simulink model "example_PV_Generator_with_Inverter"  (R2018b)
settings: Solver=ode45  StartTime=0*24*3600  StopTime=24*3600  MaxStep=60  RelTol=1e-4  EnableMultiTasking=on
undefined symbols (not defined in the file): path_carnot
libraries: carnot x4
settings Model: Creator=drhf  LastModifiedBy=drhf
settings DataIOCC: LimitDataPoints=on  SaveFormat=Array  SignalLoggingSaveFormat=ModelDataLogs
settings OptimizationCC: ExpressionDepthLimit=2147483647  LifeSpan=inf
settings DebuggingCC: UnderspecifiedInitializationDetection=Classic  MergeDetectMultiDrivingBlocksExec=none  SolverPrmCheckMsg=warning  FcnCallInpInsideContextMsg=warning  StateNameClashWarn=warning  SFUnexpectedBacktrackingDiag=warning  SFNoUnconditionalDefaultTransitionDiag=warning  SFExecutionAtInitializationDiag=none
settings HardwareCC: ProdBitPerPointer=32  ProdBitPerSizeT=32  ProdBitPerPtrDiffT=32  ProdLargestAtomicFloat=None  ProdIntDivRoundTo=Undefined  ProdEndianess=Unspecified  ProdWordSize=32  ProdHWDeviceType=32-bit Generic
settings ModelReferenceCC: PropagateSignalLabelsOutOfModel=off
settings SFSimCC: SimUseLocalCustomCode=off
settings RTWCC: RTWUseLocalCustomCode=off
settings CodeAppCC: StateflowObjectComments=on
settings GRTTargetCC: TargetLangStandard=C89/C90 (ANSI)  GeneratePreprocessorConditionals=Disable all  CombineOutputUpdateFcns=off  GRTInterface=on
settings ConfigComp: CovMetricSettings=dw  CovHtmlReporting=on  CovSaveCumulativeToWorkspaceVar=on  CovSaveSingleToWorkspaceVar=on  CovExternalEMLEnable=off

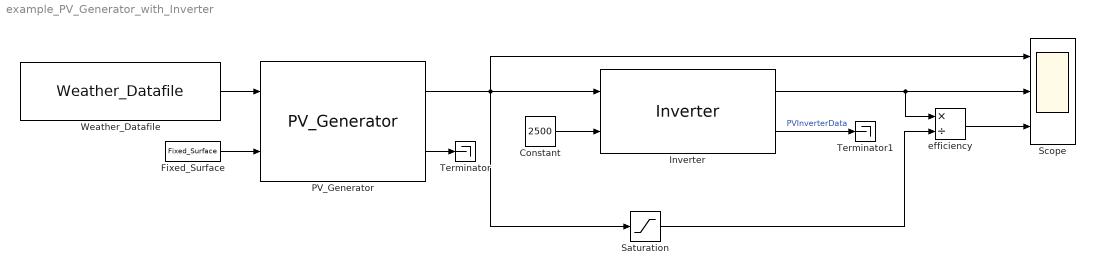
== system example_PV_Generator_with_Inverter ==
  Constant : Constant  Value=2500
  Fixed_Surface : carnot/Weather/Fixed_Surface  colangle=30  colazi=0  colrot=0
  Inverter : carnot/Source/Electric_Generator/Inverter  PathName=fullfile(path_carnot('libsl'), 'Source','Electric_Generator','Inverter','parameter_set')  FileName='SMA_SB2_5_VL40.mat'  userPath=off  userParam=off  Pacnom=2500  overload=1  PstepsEta=[0 0.1 0.2 0.25 0.3 0.5 0.75 1]  Eta=[0 0.948 0.966 0.969 0.97 0.972 0.97 0.967]  P_standby=2
  PV_Generator : carnot/Source/Electric_Generator/PV_Generator  Wp=10000  delta_Wp_K=0.0047  fgen=0.91 % 0.06 power missmatch, 0.01 diodes, 0.02 data sheet tolerance
  Saturation : Saturate  UpperLimit=inf  LowerLimit=100
  Scope : Scope  NumInputPorts=3
  Terminator : Terminator
  Terminator1 : Terminator
  Weather_Datafile : carnot/Weather/Weather_Datafile  PathName=path_carnot('data')  FileName='DE_TRY2010_04_averageYear.mat'  UserParam=off  VariableName=DE_TRY2010_04_averageYear  SampleTime=3600
  efficiency : Product  Inputs=*/
  wires:
  PV_Generator/1 -> Inverter/1, Saturation/1, Scope/1
  Inverter/1 -> efficiency/1, Scope/2
  efficiency/1 -> Scope/3
  Fixed_Surface/1 -> PV_Generator/2
  Weather_Datafile/1 -> PV_Generator/1
  Saturation/1 -> efficiency/2
  PV_Generator/2 -> Terminator/1
  Constant/1 -> Inverter/2
  Inverter/2 -> Terminator1/1  "PVInverterData"
